simulink model "fft_512pt_co_sim"  (Simulink 8.0)
settings: Solver=ode45  StartTime=0.0  StopTime=1000  RelTol=1e-3
libraries: xbsIndex_r4 x1077
(part 1 of 2)
settings Model: Creator=dell  LastModifiedBy=dell

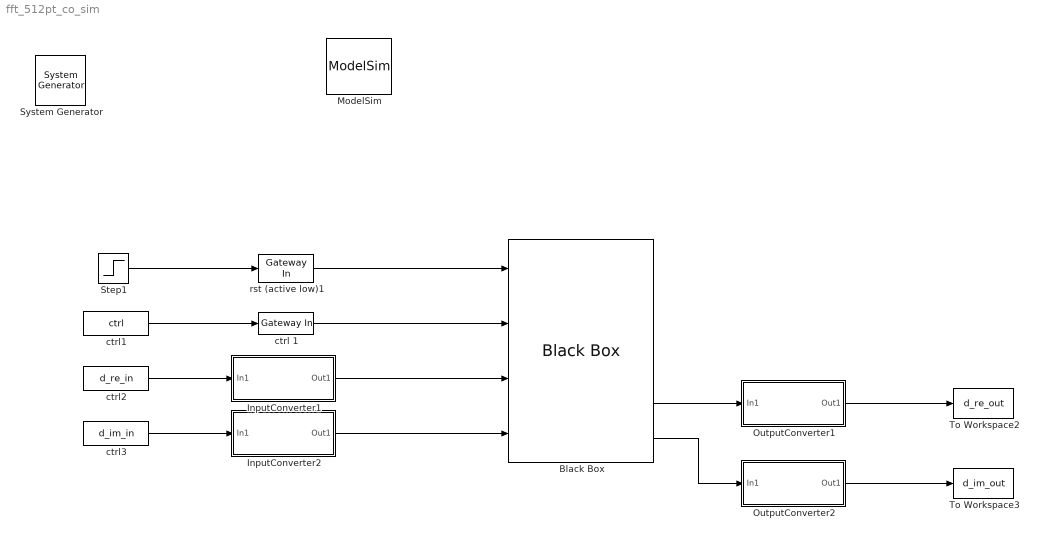
== system fft_512pt_co_sim ==
  " System Generator" : xbsIndex_r4/ System Generator  Tag=genX  xilinxfamily=Kintex7  part=xc7k325t  speed=-3  package=fbg676  synthesis_tool=XST  clock_wrapper=Clock Enables  directory=./netlist  proj_type=Project Navigator  Synth_file=XST Defaults  Impl_file=ISE Defaults  testbench=off  simulink_period=1  sysclk_period=10  dcm_input_clock_period=10  incr_netlist=off  trim_vbits=Everywhere in SubSystem  dbl_ovrd=According to Block Masks  core_generation=According to Block Masks  run_coregen=off  deprecated_control=off  eval_field=0  block_type=sysgen
  Black Box : xbsIndex_r4/Black Box  init_code=fft_pt512_config  sim_method=Inactive  verbose=off  block_type=blackbox2
  InputConverter1 : Subsystem
  InputConverter2 : Subsystem
  ModelSim : xbsIndex_r4/ModelSim  dir=./modelsim  waveform=on  leave_open=on  skip_compile=off  use_unisim=off  use_ver_xilinxcorelib=off  custom_scripts=on  post_vsim_script=./before.do  startup_timeout=40  block_type=hdlcosim
      settings: infoedit="Allow other blocks to schedule HDL co-simulation tasks.<br><br>Note that selecting \"Skip compilation\" when inappropriate can cause simulation errors and failures. Please refer to the block help for details."
  OutputConverter1 : Subsystem
  OutputConverter2 : Subsystem
  Step1 : Step  SampleTime=1
  To Workspace2 : ToWorkspace  VariableName=d_re_out  SampleTime=-1  SaveFormat=Timeseries
  To Workspace3 : ToWorkspace  VariableName=d_im_out  SampleTime=-1  SaveFormat=Timeseries
  ctrl 1 : xbsIndex_r4/Gateway In  gui_display_data_type=Boolean  arith_type=Boolean  n_bits=2  bin_pt=0  preci_type=Single  exp_width=8  frac_width=24  quantization="Round  (unbiased: +/- Inf)"  overflow=Saturate  period=1  dbl_ovrd=off  timing_constraint=None  locs_specified=off  LOCs={}  UseAsADC=off  ADCChannel='1'  inherit_from_input=off  hdl_port=on  block_type=gatewayin
      settings: xl_area=[0, 0, 0, 0, 0, 0, 0]  block_version=VER_STRING_GOES_HERE
  ctrl1 : FromWorkspace  VariableName=ctrl  SampleTime=1
  ctrl2 : FromWorkspace  VariableName=d_re_in  SampleTime=1  Interpolate=off  OutputAfterFinalValue=Setting to zero
  ctrl3 : FromWorkspace  VariableName=d_im_in  SampleTime=1  Interpolate=off  OutputAfterFinalValue=Setting to zero
  rst (active low)1 : xbsIndex_r4/Gateway In  gui_display_data_type=Boolean  arith_type=Boolean  n_bits=10  bin_pt=8  preci_type=Single  exp_width=8  frac_width=24  quantization="Round  (unbiased: +/- Inf)"  overflow=Saturate  period=1  dbl_ovrd=off  timing_constraint=None  locs_specified=off  LOCs={}  UseAsADC=off  ADCChannel='1'  inherit_from_input=off  hdl_port=on  block_type=gatewayin
      settings: xl_area=[0, 0, 0, 0, 0, 0, 0]  block_version=VER_STRING_GOES_HERE
  wires:
  Step1/1 -> rst (active low)1/1
  ctrl1/1 -> ctrl 1/1
  ctrl 1/1 -> Black Box/2
  rst (active low)1/1 -> Black Box/1
  ctrl2/1 -> InputConverter1/1(In1)
  InputConverter1/1(Out1) -> Black Box/3
  ctrl3/1 -> InputConverter2/1(In1)
  InputConverter2/1(Out1) -> Black Box/4
  Black Box/5 -> OutputConverter1/1(In1)
  OutputConverter1/1(Out1) -> To Workspace2/1
  Black Box/6 -> OutputConverter2/1(In1)
  OutputConverter2/1(Out1) -> To Workspace3/1

== system fft_512pt_co_sim/InputConverter1 ==
  In1 : Inport
  Concat : xbsIndex_r4/Concat  num_inputs=8  dbl_ovrd=off  block_type=concat
  Demux : Demux  Outputs=8
  dataconv : Subsystem
  dataconv1 : Subsystem
  dataconv13 : Subsystem
  dataconv26 : Subsystem
  dataconv28 : Subsystem
  dataconv29 : Subsystem
  dataconv3 : Subsystem
  dataconv7 : Subsystem
  Out1 : Outport
  wires:
  Demux/3 -> dataconv26/1(In1)
  Demux/7 -> dataconv28/1(In1)
  Demux/4 -> dataconv7/1(In1)
  Demux/2 -> dataconv29/1(In1)
  Demux/1 -> dataconv/1(In1)
  Demux/5 -> dataconv3/1(In1)
  Demux/6 -> dataconv13/1(In1)
  dataconv/1(Out1) -> Concat/1
  dataconv28/1(Out1) -> Concat/7
  dataconv26/1(Out1) -> Concat/3
  dataconv29/1(Out1) -> Concat/2
  dataconv13/1(Out1) -> Concat/6
  dataconv7/1(Out1) -> Concat/4
  dataconv3/1(Out1) -> Concat/5
  In1/1 -> Demux/1
  Concat/1 -> Out1/1
  Demux/8 -> dataconv1/1(In1)
  dataconv1/1(Out1) -> Concat/8

== system fft_512pt_co_sim/InputConverter2 ==
  In1 : Inport
  Concat : xbsIndex_r4/Concat  num_inputs=8  dbl_ovrd=off  block_type=concat
  Demux : Demux  Outputs=8
  dataconv : Subsystem
  dataconv1 : Subsystem
  dataconv13 : Subsystem
  dataconv26 : Subsystem
  dataconv28 : Subsystem
  dataconv29 : Subsystem
  dataconv3 : Subsystem
  dataconv7 : Subsystem
  Out1 : Outport
  wires:
  Demux/3 -> dataconv26/1(In1)
  Demux/7 -> dataconv28/1(In1)
  Demux/4 -> dataconv7/1(In1)
  Demux/2 -> dataconv29/1(In1)
  Demux/1 -> dataconv/1(In1)
  Demux/5 -> dataconv3/1(In1)
  Demux/6 -> dataconv13/1(In1)
  dataconv/1(Out1) -> Concat/1
  dataconv28/1(Out1) -> Concat/7
  dataconv26/1(Out1) -> Concat/3
  dataconv29/1(Out1) -> Concat/2
  dataconv13/1(Out1) -> Concat/6
  dataconv7/1(Out1) -> Concat/4
  dataconv3/1(Out1) -> Concat/5
  In1/1 -> Demux/1
  Concat/1 -> Out1/1
  Demux/8 -> dataconv1/1(In1)
  dataconv1/1(Out1) -> Concat/8

== system fft_512pt_co_sim/OutputConverter1 ==
  In1 : Inport
  512to64 : Subsystem
  Gateway Out{,1..3,15..18} (8 alike) : xbsIndex_r4/Gateway Out  inherit_from_input=on  hdl_port=on  timing_constraint=None  locs_specified=off  LOCs={}  UseAsDAC=off  DACChannel='1'  block_type=gatewayout
  Mux : Mux  Inputs=8
  Out1 : Outport
  wires:
  In1/1 -> 512to64/1(In1)
  512to64/2(Out3) -> Gateway Out/1
  512to64/1(Out2) -> Gateway Out15/1
  512to64/4(Out5) -> Gateway Out17/1
  512to64/3(Out4) -> Gateway Out16/1
  512to64/5(Out6) -> Gateway Out18/1
  Gateway Out15/1 -> Mux/1
  Gateway Out16/1 -> Mux/3
  Gateway Out17/1 -> Mux/4
  Gateway Out18/1 -> Mux/5
  Gateway Out/1 -> Mux/2
  Mux/1 -> Out1/1
  512to64/6(Out7) -> Gateway Out1/1
  Gateway Out1/1 -> Mux/6
  Gateway Out2/1 -> Mux/7
  512to64/7(Out8) -> Gateway Out2/1
  512to64/8(Out9) -> Gateway Out3/1
  Gateway Out3/1 -> Mux/8

== system fft_512pt_co_sim/OutputConverter2 ==
  In1 : Inport
  512to64 : Subsystem
  Gateway Out{,1..3,15..18} (8 alike) : xbsIndex_r4/Gateway Out  inherit_from_input=on  hdl_port=on  timing_constraint=None  locs_specified=off  LOCs={}  UseAsDAC=off  DACChannel='1'  block_type=gatewayout
  Mux : Mux  Inputs=8
  Out1 : Outport
  wires:
  In1/1 -> 512to64/1(In1)
  512to64/2(Out3) -> Gateway Out/1
  512to64/1(Out2) -> Gateway Out15/1
  512to64/4(Out5) -> Gateway Out17/1
  512to64/3(Out4) -> Gateway Out16/1
  512to64/5(Out6) -> Gateway Out18/1
  Gateway Out15/1 -> Mux/1
  Gateway Out16/1 -> Mux/3
  Gateway Out17/1 -> Mux/4
  Gateway Out18/1 -> Mux/5
  Gateway Out/1 -> Mux/2
  Mux/1 -> Out1/1
  512to64/6(Out7) -> Gateway Out1/1
  Gateway Out1/1 -> Mux/6
  Gateway Out2/1 -> Mux/7
  512to64/7(Out8) -> Gateway Out2/1
  512to64/8(Out9) -> Gateway Out3/1
  Gateway Out3/1 -> Mux/8

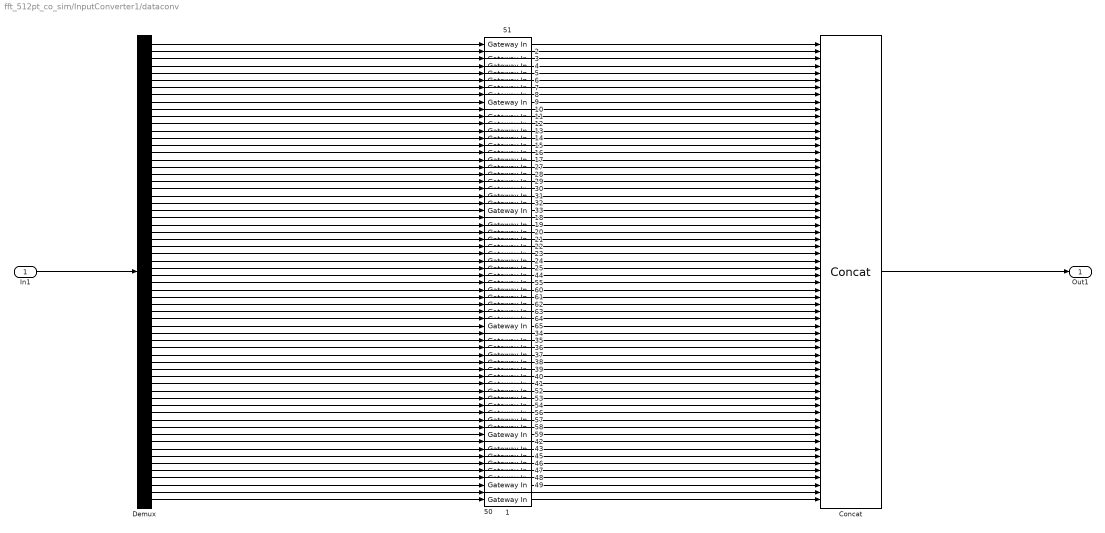
== system fft_512pt_co_sim/InputConverter1/dataconv ==
  In1 : Inport
   {1..25,27..65} (64 alike) : xbsIndex_r4/Gateway In  gui_display_data_type=Boolean  arith_type=Boolean  n_bits=16  bin_pt=14  preci_type=Single  exp_width=8  frac_width=24  quantization="Round  (unbiased: +/- Inf)"  overflow=Saturate  period=1  dbl_ovrd=off  timing_constraint=None  locs_specified=off  LOCs={}  UseAsADC=off  ADCChannel='1'  inherit_from_input=off  hdl_port=on  block_type=gatewayin
  Concat : xbsIndex_r4/Concat  num_inputs=64  dbl_ovrd=off  block_type=concat
  Demux : Demux  Outputs=64
  Out1 : Outport
  wires:
  Demux/12 -> " 12"/1
  Demux/14 -> " 14"/1
  Demux/15 -> " 15"/1
  Demux/17 -> " 17"/1
  Demux/10 -> " 10"/1
  Demux/16 -> " 16"/1
  Demux/18 -> " 27"/1
  Demux/19 -> " 28"/1
  Demux/7 -> " 7"/1
  Demux/20 -> " 29"/1
  Demux/9 -> " 9"/1
  Demux/2 -> " 2"/1
  Demux/13 -> " 13"/1
  Demux/3 -> " 3"/1
  Demux/6 -> " 6"/1
  Demux/11 -> " 11"/1
  Demux/1 -> " 51"/1
  Demux/8 -> " 8"/1
  Demux/4 -> " 4"/1
  Demux/5 -> " 5"/1
  Demux/21 -> " 30"/1
  Demux/25 -> " 18"/1
  Demux/26 -> " 19"/1
  Demux/22 -> " 31"/1
  Demux/30 -> " 23"/1
  Demux/23 -> " 32"/1
  Demux/24 -> " 33"/1
  Demux/27 -> " 20"/1
  Demux/28 -> " 21"/1
  Demux/31 -> " 24"/1
  Demux/32 -> " 25"/1
  Demux/29 -> " 22"/1
  Demux/36 -> " 61"/1
  Demux/34 -> " 55"/1
  Demux/35 -> " 60"/1
  Demux/33 -> " 44"/1
  Demux/49 -> " 52"/1
  Demux/43 -> " 36"/1
  Demux/42 -> " 35"/1
  Demux/44 -> " 37"/1
  Demux/51 -> " 54"/1
  Demux/59 -> " 46"/1
  Demux/60 -> " 47"/1
  Demux/54 -> " 58"/1
  Demux/61 -> " 48"/1
  Demux/47 -> " 40"/1
  Demux/46 -> " 39"/1
  Demux/55 -> " 59"/1
  Demux/39 -> " 64"/1
  Demux/41 -> " 34"/1
  Demux/58 -> " 45"/1
  Demux/52 -> " 56"/1
  Demux/53 -> " 57"/1
  Demux/56 -> " 42"/1
  Demux/57 -> " 43"/1
  Demux/38 -> " 63"/1
  Demux/62 -> " 49"/1
  Demux/50 -> " 53"/1
  Demux/63 -> " 1"/1
  Demux/40 -> " 65"/1
  Demux/48 -> " 41"/1
  Demux/64 -> " 50"/1
  Demux/45 -> " 38"/1
  Demux/37 -> " 62"/1
  " 13"/1 -> Concat/13
  " 11"/1 -> Concat/11
  " 16"/1 -> Concat/16
  " 15"/1 -> Concat/15
  " 10"/1 -> Concat/10
  " 14"/1 -> Concat/14
  " 12"/1 -> Concat/12
  " 17"/1 -> Concat/17
  " 2"/1 -> Concat/2
  " 3"/1 -> Concat/3
  " 7"/1 -> Concat/7
  " 6"/1 -> Concat/6
  " 9"/1 -> Concat/9
  " 8"/1 -> Concat/8
  " 42"/1 -> Concat/56
  " 35"/1 -> Concat/42
  " 43"/1 -> Concat/57
  " 40"/1 -> Concat/47
  " 36"/1 -> Concat/43
  " 34"/1 -> Concat/41
  " 37"/1 -> Concat/44
  " 38"/1 -> Concat/45
  " 41"/1 -> Concat/48
  " 39"/1 -> Concat/46
  " 52"/1 -> Concat/49
  " 56"/1 -> Concat/52
  " 49"/1 -> Concat/62
  " 1"/1 -> Concat/63
  " 44"/1 -> Concat/33
  " 55"/1 -> Concat/34
  " 54"/1 -> Concat/51
  " 53"/1 -> Concat/50
  " 48"/1 -> Concat/61
  " 46"/1 -> Concat/59
  " 45"/1 -> Concat/58
  " 47"/1 -> Concat/60
  " 63"/1 -> Concat/38
  " 62"/1 -> Concat/37
  " 64"/1 -> Concat/39
  " 60"/1 -> Concat/35
  " 65"/1 -> Concat/40
  " 59"/1 -> Concat/55
  " 58"/1 -> Concat/54
  " 57"/1 -> Concat/53
  " 61"/1 -> Concat/36
  " 19"/1 -> Concat/26
  " 20"/1 -> Concat/27
  " 21"/1 -> Concat/28
  " 22"/1 -> Concat/29
  " 23"/1 -> Concat/30
  " 18"/1 -> Concat/25
  " 24"/1 -> Concat/31
  " 25"/1 -> Concat/32
  " 28"/1 -> Concat/19
  " 27"/1 -> Concat/18
  " 30"/1 -> Concat/21
  " 29"/1 -> Concat/20
  " 31"/1 -> Concat/22
  " 32"/1 -> Concat/23
  " 33"/1 -> Concat/24
  " 4"/1 -> Concat/4
  " 5"/1 -> Concat/5
  " 50"/1 -> Concat/64
  " 51"/1 -> Concat/1
  In1/1 -> Demux/1
  Concat/1 -> Out1/1

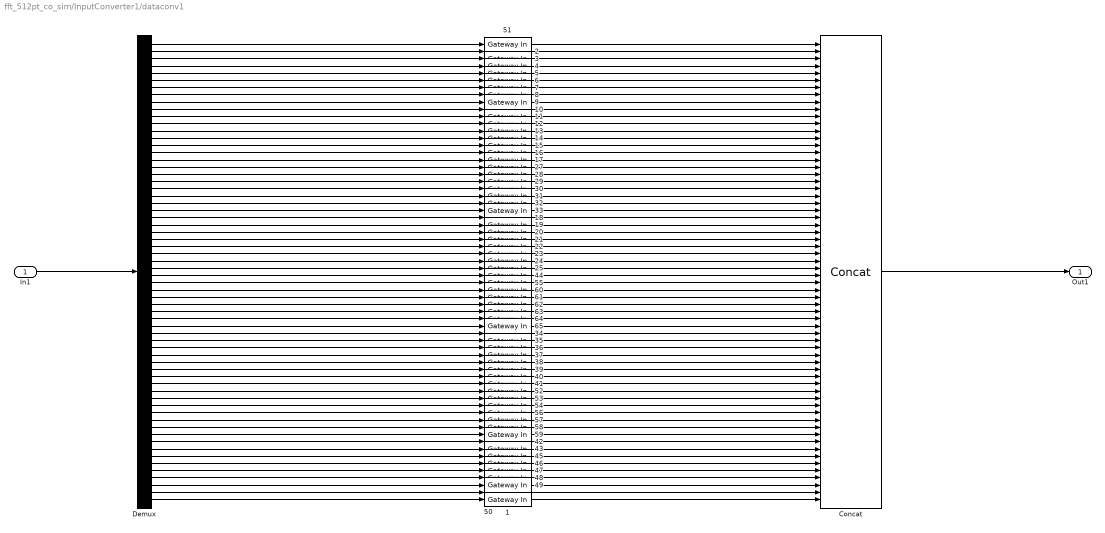
== system fft_512pt_co_sim/InputConverter1/dataconv1 ==
  In1 : Inport
   {1..25,27..65} (64 alike) : xbsIndex_r4/Gateway In  gui_display_data_type=Boolean  arith_type=Boolean  n_bits=16  bin_pt=14  preci_type=Single  exp_width=8  frac_width=24  quantization="Round  (unbiased: +/- Inf)"  overflow=Saturate  period=1  dbl_ovrd=off  timing_constraint=None  locs_specified=off  LOCs={}  UseAsADC=off  ADCChannel='1'  inherit_from_input=off  hdl_port=on  block_type=gatewayin
  Concat : xbsIndex_r4/Concat  num_inputs=64  dbl_ovrd=off  block_type=concat
  Demux : Demux  Outputs=64
  Out1 : Outport
  wires:
  Demux/12 -> " 12"/1
  Demux/14 -> " 14"/1
  Demux/15 -> " 15"/1
  Demux/17 -> " 17"/1
  Demux/10 -> " 10"/1
  Demux/16 -> " 16"/1
  Demux/18 -> " 27"/1
  Demux/19 -> " 28"/1
  Demux/7 -> " 7"/1
  Demux/20 -> " 29"/1
  Demux/9 -> " 9"/1
  Demux/2 -> " 2"/1
  Demux/13 -> " 13"/1
  Demux/3 -> " 3"/1
  Demux/6 -> " 6"/1
  Demux/11 -> " 11"/1
  Demux/1 -> " 51"/1
  Demux/8 -> " 8"/1
  Demux/4 -> " 4"/1
  Demux/5 -> " 5"/1
  Demux/21 -> " 30"/1
  Demux/25 -> " 18"/1
  Demux/26 -> " 19"/1
  Demux/22 -> " 31"/1
  Demux/30 -> " 23"/1
  Demux/23 -> " 32"/1
  Demux/24 -> " 33"/1
  Demux/27 -> " 20"/1
  Demux/28 -> " 21"/1
  Demux/31 -> " 24"/1
  Demux/32 -> " 25"/1
  Demux/29 -> " 22"/1
  Demux/36 -> " 61"/1
  Demux/34 -> " 55"/1
  Demux/35 -> " 60"/1
  Demux/33 -> " 44"/1
  Demux/49 -> " 52"/1
  Demux/43 -> " 36"/1
  Demux/42 -> " 35"/1
  Demux/44 -> " 37"/1
  Demux/51 -> " 54"/1
  Demux/59 -> " 46"/1
  Demux/60 -> " 47"/1
  Demux/54 -> " 58"/1
  Demux/61 -> " 48"/1
  Demux/47 -> " 40"/1
  Demux/46 -> " 39"/1
  Demux/55 -> " 59"/1
  Demux/39 -> " 64"/1
  Demux/41 -> " 34"/1
  Demux/58 -> " 45"/1
  Demux/52 -> " 56"/1
  Demux/53 -> " 57"/1
  Demux/56 -> " 42"/1
  Demux/57 -> " 43"/1
  Demux/38 -> " 63"/1
  Demux/62 -> " 49"/1
  Demux/50 -> " 53"/1
  Demux/63 -> " 1"/1
  Demux/40 -> " 65"/1
  Demux/48 -> " 41"/1
  Demux/64 -> " 50"/1
  Demux/45 -> " 38"/1
  Demux/37 -> " 62"/1
  " 13"/1 -> Concat/13
  " 11"/1 -> Concat/11
  " 16"/1 -> Concat/16
  " 15"/1 -> Concat/15
  " 10"/1 -> Concat/10
  " 14"/1 -> Concat/14
  " 12"/1 -> Concat/12
  " 17"/1 -> Concat/17
  " 2"/1 -> Concat/2
  " 3"/1 -> Concat/3
  " 7"/1 -> Concat/7
  " 6"/1 -> Concat/6
  " 9"/1 -> Concat/9
  " 8"/1 -> Concat/8
  " 42"/1 -> Concat/56
  " 35"/1 -> Concat/42
  " 43"/1 -> Concat/57
  " 40"/1 -> Concat/47
  " 36"/1 -> Concat/43
  " 34"/1 -> Concat/41
  " 37"/1 -> Concat/44
  " 38"/1 -> Concat/45
  " 41"/1 -> Concat/48
  " 39"/1 -> Concat/46
  " 52"/1 -> Concat/49
  " 56"/1 -> Concat/52
  " 49"/1 -> Concat/62
  " 1"/1 -> Concat/63
  " 44"/1 -> Concat/33
  " 55"/1 -> Concat/34
  " 54"/1 -> Concat/51
  " 53"/1 -> Concat/50
  " 48"/1 -> Concat/61
  " 46"/1 -> Concat/59
  " 45"/1 -> Concat/58
  " 47"/1 -> Concat/60
  " 63"/1 -> Concat/38
  " 62"/1 -> Concat/37
  " 64"/1 -> Concat/39
  " 60"/1 -> Concat/35
  " 65"/1 -> Concat/40
  " 59"/1 -> Concat/55
  " 58"/1 -> Concat/54
  " 57"/1 -> Concat/53
  " 61"/1 -> Concat/36
  " 19"/1 -> Concat/26
  " 20"/1 -> Concat/27
  " 21"/1 -> Concat/28
  " 22"/1 -> Concat/29
  " 23"/1 -> Concat/30
  " 18"/1 -> Concat/25
  " 24"/1 -> Concat/31
  " 25"/1 -> Concat/32
  " 28"/1 -> Concat/19
  " 27"/1 -> Concat/18
  " 30"/1 -> Concat/21
  " 29"/1 -> Concat/20
  " 31"/1 -> Concat/22
  " 32"/1 -> Concat/23
  " 33"/1 -> Concat/24
  " 4"/1 -> Concat/4
  " 5"/1 -> Concat/5
  " 50"/1 -> Concat/64
  " 51"/1 -> Concat/1
  In1/1 -> Demux/1
  Concat/1 -> Out1/1

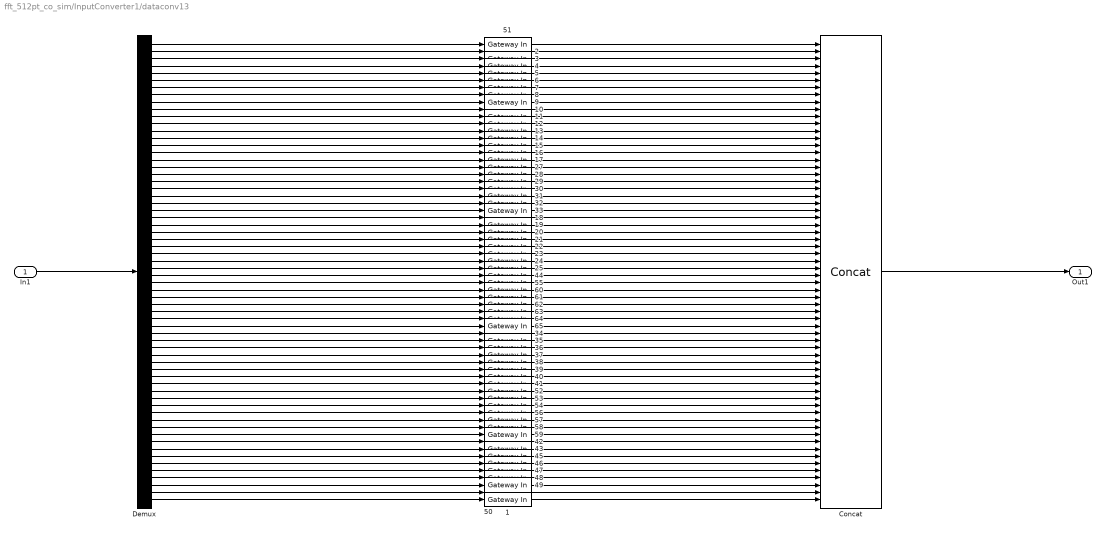
== system fft_512pt_co_sim/InputConverter1/dataconv13 ==
  In1 : Inport
   {1..25,27..65} (64 alike) : xbsIndex_r4/Gateway In  gui_display_data_type=Boolean  arith_type=Boolean  n_bits=16  bin_pt=14  preci_type=Single  exp_width=8  frac_width=24  quantization="Round  (unbiased: +/- Inf)"  overflow=Saturate  period=1  dbl_ovrd=off  timing_constraint=None  locs_specified=off  LOCs={}  UseAsADC=off  ADCChannel='1'  inherit_from_input=off  hdl_port=on  block_type=gatewayin
  Concat : xbsIndex_r4/Concat  num_inputs=64  dbl_ovrd=off  block_type=concat
  Demux : Demux  Outputs=64
  Out1 : Outport
  wires:
  Demux/12 -> " 12"/1
  Demux/14 -> " 14"/1
  Demux/15 -> " 15"/1
  Demux/17 -> " 17"/1
  Demux/10 -> " 10"/1
  Demux/16 -> " 16"/1
  Demux/18 -> " 27"/1
  Demux/19 -> " 28"/1
  Demux/7 -> " 7"/1
  Demux/20 -> " 29"/1
  Demux/9 -> " 9"/1
  Demux/2 -> " 2"/1
  Demux/13 -> " 13"/1
  Demux/3 -> " 3"/1
  Demux/6 -> " 6"/1
  Demux/11 -> " 11"/1
  Demux/1 -> " 51"/1
  Demux/8 -> " 8"/1
  Demux/4 -> " 4"/1
  Demux/5 -> " 5"/1
  Demux/21 -> " 30"/1
  Demux/25 -> " 18"/1
  Demux/26 -> " 19"/1
  Demux/22 -> " 31"/1
  Demux/30 -> " 23"/1
  Demux/23 -> " 32"/1
  Demux/24 -> " 33"/1
  Demux/27 -> " 20"/1
  Demux/28 -> " 21"/1
  Demux/31 -> " 24"/1
  Demux/32 -> " 25"/1
  Demux/29 -> " 22"/1
  Demux/36 -> " 61"/1
  Demux/34 -> " 55"/1
  Demux/35 -> " 60"/1
  Demux/33 -> " 44"/1
  Demux/49 -> " 52"/1
  Demux/43 -> " 36"/1
  Demux/42 -> " 35"/1
  Demux/44 -> " 37"/1
  Demux/51 -> " 54"/1
  Demux/59 -> " 46"/1
  Demux/60 -> " 47"/1
  Demux/54 -> " 58"/1
  Demux/61 -> " 48"/1
  Demux/47 -> " 40"/1
  Demux/46 -> " 39"/1
  Demux/55 -> " 59"/1
  Demux/39 -> " 64"/1
  Demux/41 -> " 34"/1
  Demux/58 -> " 45"/1
  Demux/52 -> " 56"/1
  Demux/53 -> " 57"/1
  Demux/56 -> " 42"/1
  Demux/57 -> " 43"/1
  Demux/38 -> " 63"/1
  Demux/62 -> " 49"/1
  Demux/50 -> " 53"/1
  Demux/63 -> " 1"/1
  Demux/40 -> " 65"/1
  Demux/48 -> " 41"/1
  Demux/64 -> " 50"/1
  Demux/45 -> " 38"/1
  Demux/37 -> " 62"/1
  " 13"/1 -> Concat/13
  " 11"/1 -> Concat/11
  " 16"/1 -> Concat/16
  " 15"/1 -> Concat/15
  " 10"/1 -> Concat/10
  " 14"/1 -> Concat/14
  " 12"/1 -> Concat/12
  " 17"/1 -> Concat/17
  " 2"/1 -> Concat/2
  " 3"/1 -> Concat/3
  " 7"/1 -> Concat/7
  " 6"/1 -> Concat/6
  " 9"/1 -> Concat/9
  " 8"/1 -> Concat/8
  " 42"/1 -> Concat/56
  " 35"/1 -> Concat/42
  " 43"/1 -> Concat/57
  " 40"/1 -> Concat/47
  " 36"/1 -> Concat/43
  " 34"/1 -> Concat/41
  " 37"/1 -> Concat/44
  " 38"/1 -> Concat/45
  " 41"/1 -> Concat/48
  " 39"/1 -> Concat/46
  " 52"/1 -> Concat/49
  " 56"/1 -> Concat/52
  " 49"/1 -> Concat/62
  " 1"/1 -> Concat/63
  " 44"/1 -> Concat/33
  " 55"/1 -> Concat/34
  " 54"/1 -> Concat/51
  " 53"/1 -> Concat/50
  " 48"/1 -> Concat/61
  " 46"/1 -> Concat/59
  " 45"/1 -> Concat/58
  " 47"/1 -> Concat/60
  " 63"/1 -> Concat/38
  " 62"/1 -> Concat/37
  " 64"/1 -> Concat/39
  " 60"/1 -> Concat/35
  " 65"/1 -> Concat/40
  " 59"/1 -> Concat/55
  " 58"/1 -> Concat/54
  " 57"/1 -> Concat/53
  " 61"/1 -> Concat/36
  " 19"/1 -> Concat/26
  " 20"/1 -> Concat/27
  " 21"/1 -> Concat/28
  " 22"/1 -> Concat/29
  " 23"/1 -> Concat/30
  " 18"/1 -> Concat/25
  " 24"/1 -> Concat/31
  " 25"/1 -> Concat/32
  " 28"/1 -> Concat/19
  " 27"/1 -> Concat/18
  " 30"/1 -> Concat/21
  " 29"/1 -> Concat/20
  " 31"/1 -> Concat/22
  " 32"/1 -> Concat/23
  " 33"/1 -> Concat/24
  " 4"/1 -> Concat/4
  " 5"/1 -> Concat/5
  " 50"/1 -> Concat/64
  " 51"/1 -> Concat/1
  In1/1 -> Demux/1
  Concat/1 -> Out1/1

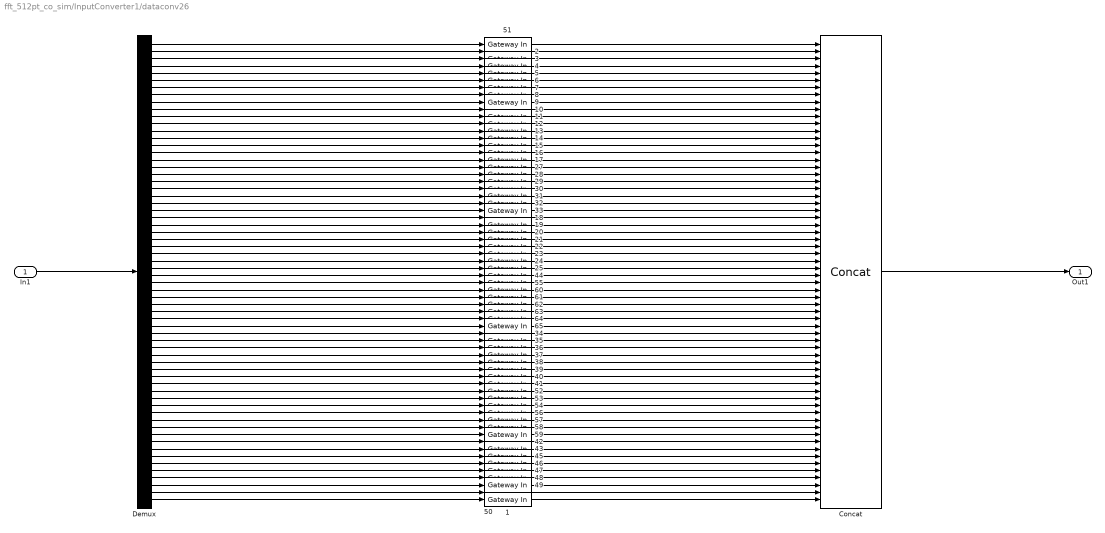
== system fft_512pt_co_sim/InputConverter1/dataconv26 ==
  In1 : Inport
   {1..25,27..65} (64 alike) : xbsIndex_r4/Gateway In  gui_display_data_type=Boolean  arith_type=Boolean  n_bits=16  bin_pt=14  preci_type=Single  exp_width=8  frac_width=24  quantization="Round  (unbiased: +/- Inf)"  overflow=Saturate  period=1  dbl_ovrd=off  timing_constraint=None  locs_specified=off  LOCs={}  UseAsADC=off  ADCChannel='1'  inherit_from_input=off  hdl_port=on  block_type=gatewayin
  Concat : xbsIndex_r4/Concat  num_inputs=64  dbl_ovrd=off  block_type=concat
  Demux : Demux  Outputs=64
  Out1 : Outport
  wires:
  Demux/12 -> " 12"/1
  Demux/14 -> " 14"/1
  Demux/15 -> " 15"/1
  Demux/17 -> " 17"/1
  Demux/10 -> " 10"/1
  Demux/16 -> " 16"/1
  Demux/18 -> " 27"/1
  Demux/19 -> " 28"/1
  Demux/7 -> " 7"/1
  Demux/20 -> " 29"/1
  Demux/9 -> " 9"/1
  Demux/2 -> " 2"/1
  Demux/13 -> " 13"/1
  Demux/3 -> " 3"/1
  Demux/6 -> " 6"/1
  Demux/11 -> " 11"/1
  Demux/1 -> " 51"/1
  Demux/8 -> " 8"/1
  Demux/4 -> " 4"/1
  Demux/5 -> " 5"/1
  Demux/21 -> " 30"/1
  Demux/25 -> " 18"/1
  Demux/26 -> " 19"/1
  Demux/22 -> " 31"/1
  Demux/30 -> " 23"/1
  Demux/23 -> " 32"/1
  Demux/24 -> " 33"/1
  Demux/27 -> " 20"/1
  Demux/28 -> " 21"/1
  Demux/31 -> " 24"/1
  Demux/32 -> " 25"/1
  Demux/29 -> " 22"/1
  Demux/36 -> " 61"/1
  Demux/34 -> " 55"/1
  Demux/35 -> " 60"/1
  Demux/33 -> " 44"/1
  Demux/49 -> " 52"/1
  Demux/43 -> " 36"/1
  Demux/42 -> " 35"/1
  Demux/44 -> " 37"/1
  Demux/51 -> " 54"/1
  Demux/59 -> " 46"/1
  Demux/60 -> " 47"/1
  Demux/54 -> " 58"/1
  Demux/61 -> " 48"/1
  Demux/47 -> " 40"/1
  Demux/46 -> " 39"/1
  Demux/55 -> " 59"/1
  Demux/39 -> " 64"/1
  Demux/41 -> " 34"/1
  Demux/58 -> " 45"/1
  Demux/52 -> " 56"/1
  Demux/53 -> " 57"/1
  Demux/56 -> " 42"/1
  Demux/57 -> " 43"/1
  Demux/38 -> " 63"/1
  Demux/62 -> " 49"/1
  Demux/50 -> " 53"/1
  Demux/63 -> " 1"/1
  Demux/40 -> " 65"/1
  Demux/48 -> " 41"/1
  Demux/64 -> " 50"/1
  Demux/45 -> " 38"/1
  Demux/37 -> " 62"/1
  " 13"/1 -> Concat/13
  " 11"/1 -> Concat/11
  " 16"/1 -> Concat/16
  " 15"/1 -> Concat/15
  " 10"/1 -> Concat/10
  " 14"/1 -> Concat/14
  " 12"/1 -> Concat/12
  " 17"/1 -> Concat/17
  " 2"/1 -> Concat/2
  " 3"/1 -> Concat/3
  " 7"/1 -> Concat/7
  " 6"/1 -> Concat/6
  " 9"/1 -> Concat/9
  " 8"/1 -> Concat/8
  " 42"/1 -> Concat/56
  " 35"/1 -> Concat/42
  " 43"/1 -> Concat/57
  " 40"/1 -> Concat/47
  " 36"/1 -> Concat/43
  " 34"/1 -> Concat/41
  " 37"/1 -> Concat/44
  " 38"/1 -> Concat/45
  " 41"/1 -> Concat/48
  " 39"/1 -> Concat/46
  " 52"/1 -> Concat/49
  " 56"/1 -> Concat/52
  " 49"/1 -> Concat/62
  " 1"/1 -> Concat/63
  " 44"/1 -> Concat/33
  " 55"/1 -> Concat/34
  " 54"/1 -> Concat/51
  " 53"/1 -> Concat/50
  " 48"/1 -> Concat/61
  " 46"/1 -> Concat/59
  " 45"/1 -> Concat/58
  " 47"/1 -> Concat/60
  " 63"/1 -> Concat/38
  " 62"/1 -> Concat/37
  " 64"/1 -> Concat/39
  " 60"/1 -> Concat/35
  " 65"/1 -> Concat/40
  " 59"/1 -> Concat/55
  " 58"/1 -> Concat/54
  " 57"/1 -> Concat/53
  " 61"/1 -> Concat/36
  " 19"/1 -> Concat/26
  " 20"/1 -> Concat/27
  " 21"/1 -> Concat/28
  " 22"/1 -> Concat/29
  " 23"/1 -> Concat/30
  " 18"/1 -> Concat/25
  " 24"/1 -> Concat/31
  " 25"/1 -> Concat/32
  " 28"/1 -> Concat/19
  " 27"/1 -> Concat/18
  " 30"/1 -> Concat/21
  " 29"/1 -> Concat/20
  " 31"/1 -> Concat/22
  " 32"/1 -> Concat/23
  " 33"/1 -> Concat/24
  " 4"/1 -> Concat/4
  " 5"/1 -> Concat/5
  " 50"/1 -> Concat/64
  " 51"/1 -> Concat/1
  In1/1 -> Demux/1
  Concat/1 -> Out1/1

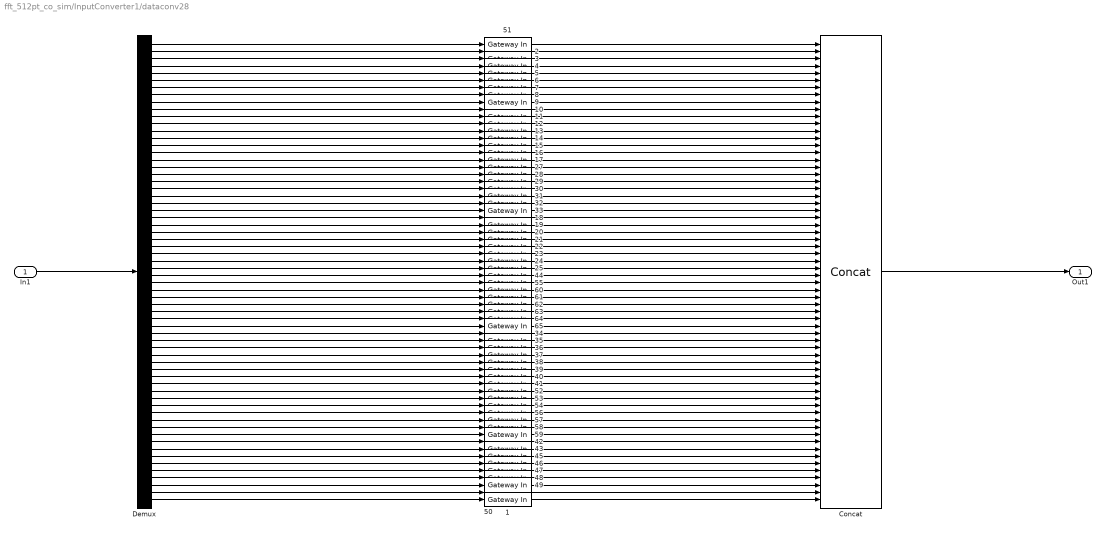
== system fft_512pt_co_sim/InputConverter1/dataconv28 ==
  In1 : Inport
   {1..25,27..65} (64 alike) : xbsIndex_r4/Gateway In  gui_display_data_type=Boolean  arith_type=Boolean  n_bits=16  bin_pt=14  preci_type=Single  exp_width=8  frac_width=24  quantization="Round  (unbiased: +/- Inf)"  overflow=Saturate  period=1  dbl_ovrd=off  timing_constraint=None  locs_specified=off  LOCs={}  UseAsADC=off  ADCChannel='1'  inherit_from_input=off  hdl_port=on  block_type=gatewayin
  Concat : xbsIndex_r4/Concat  num_inputs=64  dbl_ovrd=off  block_type=concat
  Demux : Demux  Outputs=64
  Out1 : Outport
  wires:
  Demux/12 -> " 12"/1
  Demux/14 -> " 14"/1
  Demux/15 -> " 15"/1
  Demux/17 -> " 17"/1
  Demux/10 -> " 10"/1
  Demux/16 -> " 16"/1
  Demux/18 -> " 27"/1
  Demux/19 -> " 28"/1
  Demux/7 -> " 7"/1
  Demux/20 -> " 29"/1
  Demux/9 -> " 9"/1
  Demux/2 -> " 2"/1
  Demux/13 -> " 13"/1
  Demux/3 -> " 3"/1
  Demux/6 -> " 6"/1
  Demux/11 -> " 11"/1
  Demux/1 -> " 51"/1
  Demux/8 -> " 8"/1
  Demux/4 -> " 4"/1
  Demux/5 -> " 5"/1
  Demux/21 -> " 30"/1
  Demux/25 -> " 18"/1
  Demux/26 -> " 19"/1
  Demux/22 -> " 31"/1
  Demux/30 -> " 23"/1
  Demux/23 -> " 32"/1
  Demux/24 -> " 33"/1
  Demux/27 -> " 20"/1
  Demux/28 -> " 21"/1
  Demux/31 -> " 24"/1
  Demux/32 -> " 25"/1
  Demux/29 -> " 22"/1
  Demux/36 -> " 61"/1
  Demux/34 -> " 55"/1
  Demux/35 -> " 60"/1
  Demux/33 -> " 44"/1
  Demux/49 -> " 52"/1
  Demux/43 -> " 36"/1
  Demux/42 -> " 35"/1
  Demux/44 -> " 37"/1
  Demux/51 -> " 54"/1
  Demux/59 -> " 46"/1
  Demux/60 -> " 47"/1
  Demux/54 -> " 58"/1
  Demux/61 -> " 48"/1
  Demux/47 -> " 40"/1
  Demux/46 -> " 39"/1
  Demux/55 -> " 59"/1
  Demux/39 -> " 64"/1
  Demux/41 -> " 34"/1
  Demux/58 -> " 45"/1
  Demux/52 -> " 56"/1
  Demux/53 -> " 57"/1
  Demux/56 -> " 42"/1
  Demux/57 -> " 43"/1
  Demux/38 -> " 63"/1
  Demux/62 -> " 49"/1
  Demux/50 -> " 53"/1
  Demux/63 -> " 1"/1
  Demux/40 -> " 65"/1
  Demux/48 -> " 41"/1
  Demux/64 -> " 50"/1
  Demux/45 -> " 38"/1
  Demux/37 -> " 62"/1
  " 13"/1 -> Concat/13
  " 11"/1 -> Concat/11
  " 16"/1 -> Concat/16
  " 15"/1 -> Concat/15
  " 10"/1 -> Concat/10
  " 14"/1 -> Concat/14
  " 12"/1 -> Concat/12
  " 17"/1 -> Concat/17
  " 2"/1 -> Concat/2
  " 3"/1 -> Concat/3
  " 7"/1 -> Concat/7
  " 6"/1 -> Concat/6
  " 9"/1 -> Concat/9
  " 8"/1 -> Concat/8
  " 42"/1 -> Concat/56
  " 35"/1 -> Concat/42
  " 43"/1 -> Concat/57
  " 40"/1 -> Concat/47
  " 36"/1 -> Concat/43
  " 34"/1 -> Concat/41
  " 37"/1 -> Concat/44
  " 38"/1 -> Concat/45
  " 41"/1 -> Concat/48
  " 39"/1 -> Concat/46
  " 52"/1 -> Concat/49
  " 56"/1 -> Concat/52
  " 49"/1 -> Concat/62
  " 1"/1 -> Concat/63
  " 44"/1 -> Concat/33
  " 55"/1 -> Concat/34
  " 54"/1 -> Concat/51
  " 53"/1 -> Concat/50
  " 48"/1 -> Concat/61
  " 46"/1 -> Concat/59
  " 45"/1 -> Concat/58
  " 47"/1 -> Concat/60
  " 63"/1 -> Concat/38
  " 62"/1 -> Concat/37
  " 64"/1 -> Concat/39
  " 60"/1 -> Concat/35
  " 65"/1 -> Concat/40
  " 59"/1 -> Concat/55
  " 58"/1 -> Concat/54
  " 57"/1 -> Concat/53
  " 61"/1 -> Concat/36
  " 19"/1 -> Concat/26
  " 20"/1 -> Concat/27
  " 21"/1 -> Concat/28
  " 22"/1 -> Concat/29
  " 23"/1 -> Concat/30
  " 18"/1 -> Concat/25
  " 24"/1 -> Concat/31
  " 25"/1 -> Concat/32
  " 28"/1 -> Concat/19
  " 27"/1 -> Concat/18
  " 30"/1 -> Concat/21
  " 29"/1 -> Concat/20
  " 31"/1 -> Concat/22
  " 32"/1 -> Concat/23
  " 33"/1 -> Concat/24
  " 4"/1 -> Concat/4
  " 5"/1 -> Concat/5
  " 50"/1 -> Concat/64
  " 51"/1 -> Concat/1
  In1/1 -> Demux/1
  Concat/1 -> Out1/1

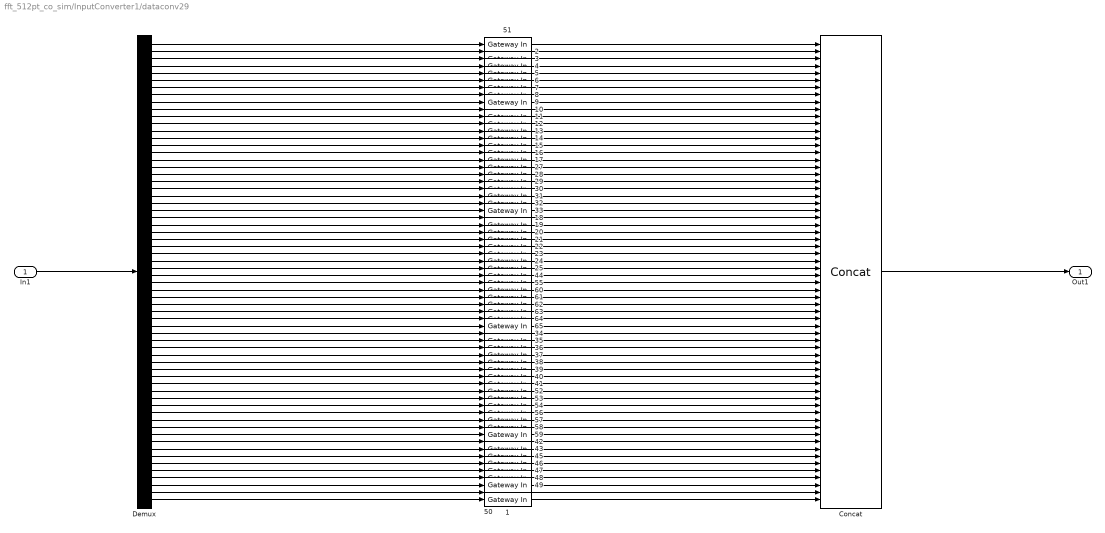
== system fft_512pt_co_sim/InputConverter1/dataconv29 ==
  In1 : Inport
   {1..25,27..65} (64 alike) : xbsIndex_r4/Gateway In  gui_display_data_type=Boolean  arith_type=Boolean  n_bits=16  bin_pt=14  preci_type=Single  exp_width=8  frac_width=24  quantization="Round  (unbiased: +/- Inf)"  overflow=Saturate  period=1  dbl_ovrd=off  timing_constraint=None  locs_specified=off  LOCs={}  UseAsADC=off  ADCChannel='1'  inherit_from_input=off  hdl_port=on  block_type=gatewayin
  Concat : xbsIndex_r4/Concat  num_inputs=64  dbl_ovrd=off  block_type=concat
  Demux : Demux  Outputs=64
  Out1 : Outport
  wires:
  Demux/12 -> " 12"/1
  Demux/14 -> " 14"/1
  Demux/15 -> " 15"/1
  Demux/17 -> " 17"/1
  Demux/10 -> " 10"/1
  Demux/16 -> " 16"/1
  Demux/18 -> " 27"/1
  Demux/19 -> " 28"/1
  Demux/7 -> " 7"/1
  Demux/20 -> " 29"/1
  Demux/9 -> " 9"/1
  Demux/2 -> " 2"/1
  Demux/13 -> " 13"/1
  Demux/3 -> " 3"/1
  Demux/6 -> " 6"/1
  Demux/11 -> " 11"/1
  Demux/1 -> " 51"/1
  Demux/8 -> " 8"/1
  Demux/4 -> " 4"/1
  Demux/5 -> " 5"/1
  Demux/21 -> " 30"/1
  Demux/25 -> " 18"/1
  Demux/26 -> " 19"/1
  Demux/22 -> " 31"/1
  Demux/30 -> " 23"/1
  Demux/23 -> " 32"/1
  Demux/24 -> " 33"/1
  Demux/27 -> " 20"/1
  Demux/28 -> " 21"/1
  Demux/31 -> " 24"/1
  Demux/32 -> " 25"/1
  Demux/29 -> " 22"/1
  Demux/36 -> " 61"/1
  Demux/34 -> " 55"/1
  Demux/35 -> " 60"/1
  Demux/33 -> " 44"/1
  Demux/49 -> " 52"/1
  Demux/43 -> " 36"/1
  Demux/42 -> " 35"/1
  Demux/44 -> " 37"/1
  Demux/51 -> " 54"/1
  Demux/59 -> " 46"/1
  Demux/60 -> " 47"/1
  Demux/54 -> " 58"/1
  Demux/61 -> " 48"/1
  Demux/47 -> " 40"/1
  Demux/46 -> " 39"/1
  Demux/55 -> " 59"/1
  Demux/39 -> " 64"/1
  Demux/41 -> " 34"/1
  Demux/58 -> " 45"/1
  Demux/52 -> " 56"/1
  Demux/53 -> " 57"/1
  Demux/56 -> " 42"/1
  Demux/57 -> " 43"/1
  Demux/38 -> " 63"/1
  Demux/62 -> " 49"/1
  Demux/50 -> " 53"/1
  Demux/63 -> " 1"/1
  Demux/40 -> " 65"/1
  Demux/48 -> " 41"/1
  Demux/64 -> " 50"/1
  Demux/45 -> " 38"/1
  Demux/37 -> " 62"/1
  " 13"/1 -> Concat/13
  " 11"/1 -> Concat/11
  " 16"/1 -> Concat/16
  " 15"/1 -> Concat/15
  " 10"/1 -> Concat/10
  " 14"/1 -> Concat/14
  " 12"/1 -> Concat/12
  " 17"/1 -> Concat/17
  " 2"/1 -> Concat/2
  " 3"/1 -> Concat/3
  " 7"/1 -> Concat/7
  " 6"/1 -> Concat/6
  " 9"/1 -> Concat/9
  " 8"/1 -> Concat/8
  " 42"/1 -> Concat/56
  " 35"/1 -> Concat/42
  " 43"/1 -> Concat/57
  " 40"/1 -> Concat/47
  " 36"/1 -> Concat/43
  " 34"/1 -> Concat/41
  " 37"/1 -> Concat/44
  " 38"/1 -> Concat/45
  " 41"/1 -> Concat/48
  " 39"/1 -> Concat/46
  " 52"/1 -> Concat/49
  " 56"/1 -> Concat/52
  " 49"/1 -> Concat/62
  " 1"/1 -> Concat/63
  " 44"/1 -> Concat/33
  " 55"/1 -> Concat/34
  " 54"/1 -> Concat/51
  " 53"/1 -> Concat/50
  " 48"/1 -> Concat/61
  " 46"/1 -> Concat/59
  " 45"/1 -> Concat/58
  " 47"/1 -> Concat/60
  " 63"/1 -> Concat/38
  " 62"/1 -> Concat/37
  " 64"/1 -> Concat/39
  " 60"/1 -> Concat/35
  " 65"/1 -> Concat/40
  " 59"/1 -> Concat/55
  " 58"/1 -> Concat/54
  " 57"/1 -> Concat/53
  " 61"/1 -> Concat/36
  " 19"/1 -> Concat/26
  " 20"/1 -> Concat/27
  " 21"/1 -> Concat/28
  " 22"/1 -> Concat/29
  " 23"/1 -> Concat/30
  " 18"/1 -> Concat/25
  " 24"/1 -> Concat/31
  " 25"/1 -> Concat/32
  " 28"/1 -> Concat/19
  " 27"/1 -> Concat/18
  " 30"/1 -> Concat/21
  " 29"/1 -> Concat/20
  " 31"/1 -> Concat/22
  " 32"/1 -> Concat/23
  " 33"/1 -> Concat/24
  " 4"/1 -> Concat/4
  " 5"/1 -> Concat/5
  " 50"/1 -> Concat/64
  " 51"/1 -> Concat/1
  In1/1 -> Demux/1
  Concat/1 -> Out1/1

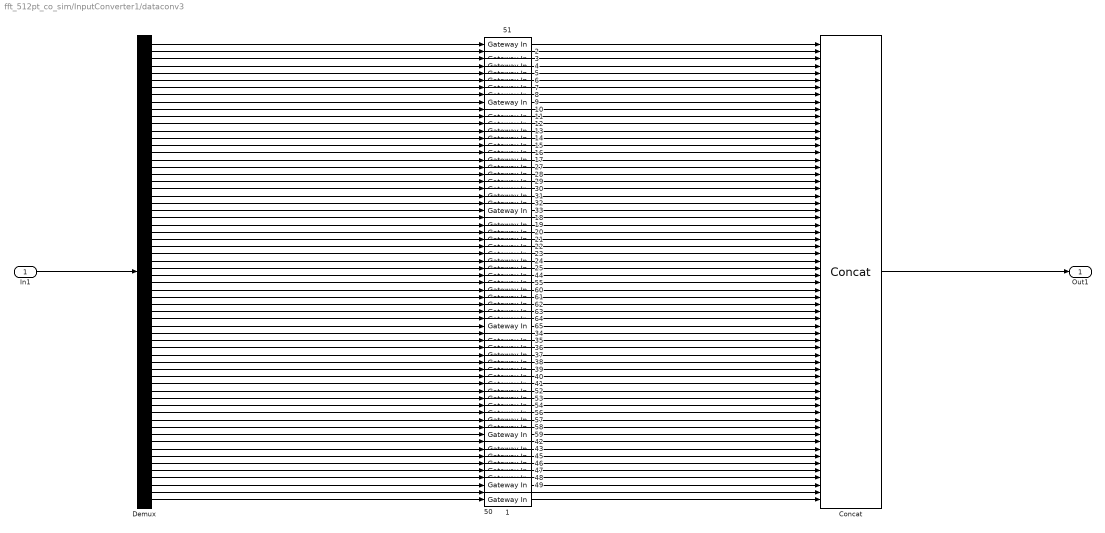
== system fft_512pt_co_sim/InputConverter1/dataconv3 ==
  In1 : Inport
   {1..25,27..65} (64 alike) : xbsIndex_r4/Gateway In  gui_display_data_type=Boolean  arith_type=Boolean  n_bits=16  bin_pt=14  preci_type=Single  exp_width=8  frac_width=24  quantization="Round  (unbiased: +/- Inf)"  overflow=Saturate  period=1  dbl_ovrd=off  timing_constraint=None  locs_specified=off  LOCs={}  UseAsADC=off  ADCChannel='1'  inherit_from_input=off  hdl_port=on  block_type=gatewayin
  Concat : xbsIndex_r4/Concat  num_inputs=64  dbl_ovrd=off  block_type=concat
  Demux : Demux  Outputs=64
  Out1 : Outport
  wires:
  Demux/12 -> " 12"/1
  Demux/14 -> " 14"/1
  Demux/15 -> " 15"/1
  Demux/17 -> " 17"/1
  Demux/10 -> " 10"/1
  Demux/16 -> " 16"/1
  Demux/18 -> " 27"/1
  Demux/19 -> " 28"/1
  Demux/7 -> " 7"/1
  Demux/20 -> " 29"/1
  Demux/9 -> " 9"/1
  Demux/2 -> " 2"/1
  Demux/13 -> " 13"/1
  Demux/3 -> " 3"/1
  Demux/6 -> " 6"/1
  Demux/11 -> " 11"/1
  Demux/1 -> " 51"/1
  Demux/8 -> " 8"/1
  Demux/4 -> " 4"/1
  Demux/5 -> " 5"/1
  Demux/21 -> " 30"/1
  Demux/25 -> " 18"/1
  Demux/26 -> " 19"/1
  Demux/22 -> " 31"/1
  Demux/30 -> " 23"/1
  Demux/23 -> " 32"/1
  Demux/24 -> " 33"/1
  Demux/27 -> " 20"/1
  Demux/28 -> " 21"/1
  Demux/31 -> " 24"/1
  Demux/32 -> " 25"/1
  Demux/29 -> " 22"/1
  Demux/36 -> " 61"/1
  Demux/34 -> " 55"/1
  Demux/35 -> " 60"/1
  Demux/33 -> " 44"/1
  Demux/49 -> " 52"/1
  Demux/43 -> " 36"/1
  Demux/42 -> " 35"/1
  Demux/44 -> " 37"/1
  Demux/51 -> " 54"/1
  Demux/59 -> " 46"/1
  Demux/60 -> " 47"/1
  Demux/54 -> " 58"/1
  Demux/61 -> " 48"/1
  Demux/47 -> " 40"/1
  Demux/46 -> " 39"/1
  Demux/55 -> " 59"/1
  Demux/39 -> " 64"/1
  Demux/41 -> " 34"/1
  Demux/58 -> " 45"/1
  Demux/52 -> " 56"/1
  Demux/53 -> " 57"/1
  Demux/56 -> " 42"/1
  Demux/57 -> " 43"/1
  Demux/38 -> " 63"/1
  Demux/62 -> " 49"/1
  Demux/50 -> " 53"/1
  Demux/63 -> " 1"/1
  Demux/40 -> " 65"/1
  Demux/48 -> " 41"/1
  Demux/64 -> " 50"/1
  Demux/45 -> " 38"/1
  Demux/37 -> " 62"/1
  " 13"/1 -> Concat/13
  " 11"/1 -> Concat/11
  " 16"/1 -> Concat/16
  " 15"/1 -> Concat/15
  " 10"/1 -> Concat/10
  " 14"/1 -> Concat/14
  " 12"/1 -> Concat/12
  " 17"/1 -> Concat/17
  " 2"/1 -> Concat/2
  " 3"/1 -> Concat/3
  " 7"/1 -> Concat/7
  " 6"/1 -> Concat/6
  " 9"/1 -> Concat/9
  " 8"/1 -> Concat/8
  " 42"/1 -> Concat/56
  " 35"/1 -> Concat/42
  " 43"/1 -> Concat/57
  " 40"/1 -> Concat/47
  " 36"/1 -> Concat/43
  " 34"/1 -> Concat/41
  " 37"/1 -> Concat/44
  " 38"/1 -> Concat/45
  " 41"/1 -> Concat/48
  " 39"/1 -> Concat/46
  " 52"/1 -> Concat/49
  " 56"/1 -> Concat/52
  " 49"/1 -> Concat/62
  " 1"/1 -> Concat/63
  " 44"/1 -> Concat/33
  " 55"/1 -> Concat/34
  " 54"/1 -> Concat/51
  " 53"/1 -> Concat/50
  " 48"/1 -> Concat/61
  " 46"/1 -> Concat/59
  " 45"/1 -> Concat/58
  " 47"/1 -> Concat/60
  " 63"/1 -> Concat/38
  " 62"/1 -> Concat/37
  " 64"/1 -> Concat/39
  " 60"/1 -> Concat/35
  " 65"/1 -> Concat/40
  " 59"/1 -> Concat/55
  " 58"/1 -> Concat/54
  " 57"/1 -> Concat/53
  " 61"/1 -> Concat/36
  " 19"/1 -> Concat/26
  " 20"/1 -> Concat/27
  " 21"/1 -> Concat/28
  " 22"/1 -> Concat/29
  " 23"/1 -> Concat/30
  " 18"/1 -> Concat/25
  " 24"/1 -> Concat/31
  " 25"/1 -> Concat/32
  " 28"/1 -> Concat/19
  " 27"/1 -> Concat/18
  " 30"/1 -> Concat/21
  " 29"/1 -> Concat/20
  " 31"/1 -> Concat/22
  " 32"/1 -> Concat/23
  " 33"/1 -> Concat/24
  " 4"/1 -> Concat/4
  " 5"/1 -> Concat/5
  " 50"/1 -> Concat/64
  " 51"/1 -> Concat/1
  In1/1 -> Demux/1
  Concat/1 -> Out1/1

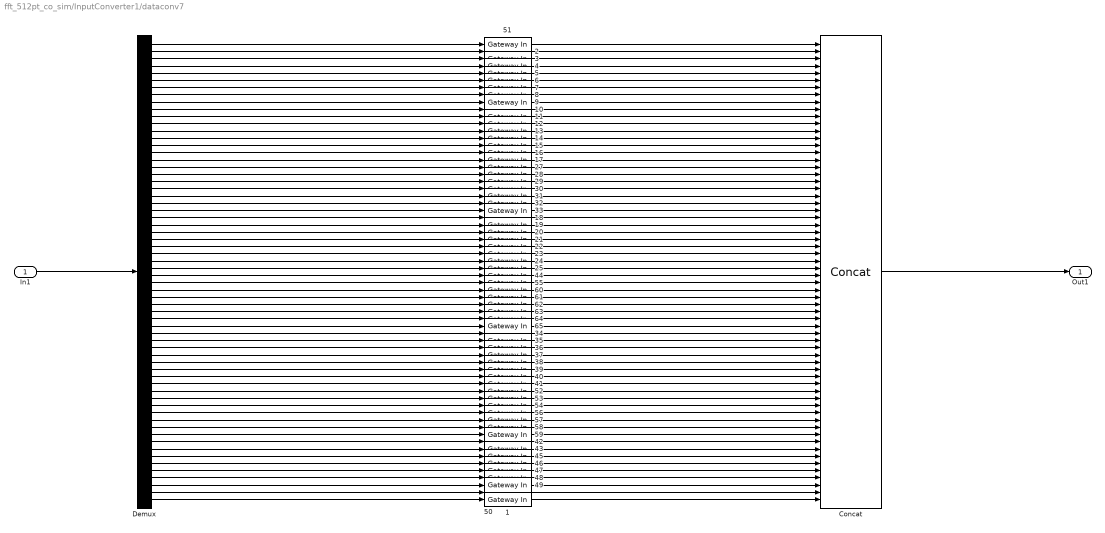
== system fft_512pt_co_sim/InputConverter1/dataconv7 ==
  In1 : Inport
   {1..25,27..65} (64 alike) : xbsIndex_r4/Gateway In  gui_display_data_type=Boolean  arith_type=Boolean  n_bits=16  bin_pt=14  preci_type=Single  exp_width=8  frac_width=24  quantization="Round  (unbiased: +/- Inf)"  overflow=Saturate  period=1  dbl_ovrd=off  timing_constraint=None  locs_specified=off  LOCs={}  UseAsADC=off  ADCChannel='1'  inherit_from_input=off  hdl_port=on  block_type=gatewayin
  Concat : xbsIndex_r4/Concat  num_inputs=64  dbl_ovrd=off  block_type=concat
  Demux : Demux  Outputs=64
  Out1 : Outport
  wires:
  Demux/12 -> " 12"/1
  Demux/14 -> " 14"/1
  Demux/15 -> " 15"/1
  Demux/17 -> " 17"/1
  Demux/10 -> " 10"/1
  Demux/16 -> " 16"/1
  Demux/18 -> " 27"/1
  Demux/19 -> " 28"/1
  Demux/7 -> " 7"/1
  Demux/20 -> " 29"/1
  Demux/9 -> " 9"/1
  Demux/2 -> " 2"/1
  Demux/13 -> " 13"/1
  Demux/3 -> " 3"/1
  Demux/6 -> " 6"/1
  Demux/11 -> " 11"/1
  Demux/1 -> " 51"/1
  Demux/8 -> " 8"/1
  Demux/4 -> " 4"/1
  Demux/5 -> " 5"/1
  Demux/21 -> " 30"/1
  Demux/25 -> " 18"/1
  Demux/26 -> " 19"/1
  Demux/22 -> " 31"/1
  Demux/30 -> " 23"/1
  Demux/23 -> " 32"/1
  Demux/24 -> " 33"/1
  Demux/27 -> " 20"/1
  Demux/28 -> " 21"/1
  Demux/31 -> " 24"/1
  Demux/32 -> " 25"/1
  Demux/29 -> " 22"/1
  Demux/36 -> " 61"/1
  Demux/34 -> " 55"/1
  Demux/35 -> " 60"/1
  Demux/33 -> " 44"/1
  Demux/49 -> " 52"/1
  Demux/43 -> " 36"/1
  Demux/42 -> " 35"/1
  Demux/44 -> " 37"/1
  Demux/51 -> " 54"/1
  Demux/59 -> " 46"/1
  Demux/60 -> " 47"/1
  Demux/54 -> " 58"/1
  Demux/61 -> " 48"/1
  Demux/47 -> " 40"/1
  Demux/46 -> " 39"/1
  Demux/55 -> " 59"/1
  Demux/39 -> " 64"/1
  Demux/41 -> " 34"/1
  Demux/58 -> " 45"/1
  Demux/52 -> " 56"/1
  Demux/53 -> " 57"/1
  Demux/56 -> " 42"/1
  Demux/57 -> " 43"/1
  Demux/38 -> " 63"/1
  Demux/62 -> " 49"/1
  Demux/50 -> " 53"/1
  Demux/63 -> " 1"/1
  Demux/40 -> " 65"/1
  Demux/48 -> " 41"/1
  Demux/64 -> " 50"/1
  Demux/45 -> " 38"/1
  Demux/37 -> " 62"/1
  " 13"/1 -> Concat/13
  " 11"/1 -> Concat/11
  " 16"/1 -> Concat/16
  " 15"/1 -> Concat/15
  " 10"/1 -> Concat/10
  " 14"/1 -> Concat/14
  " 12"/1 -> Concat/12
  " 17"/1 -> Concat/17
  " 2"/1 -> Concat/2
  " 3"/1 -> Concat/3
  " 7"/1 -> Concat/7
  " 6"/1 -> Concat/6
  " 9"/1 -> Concat/9
  " 8"/1 -> Concat/8
  " 42"/1 -> Concat/56
  " 35"/1 -> Concat/42
  " 43"/1 -> Concat/57
  " 40"/1 -> Concat/47
  " 36"/1 -> Concat/43
  " 34"/1 -> Concat/41
  " 37"/1 -> Concat/44
  " 38"/1 -> Concat/45
  " 41"/1 -> Concat/48
  " 39"/1 -> Concat/46
  " 52"/1 -> Concat/49
  " 56"/1 -> Concat/52
  " 49"/1 -> Concat/62
  " 1"/1 -> Concat/63
  " 44"/1 -> Concat/33
  " 55"/1 -> Concat/34
  " 54"/1 -> Concat/51
  " 53"/1 -> Concat/50
  " 48"/1 -> Concat/61
  " 46"/1 -> Concat/59
  " 45"/1 -> Concat/58
  " 47"/1 -> Concat/60
  " 63"/1 -> Concat/38
  " 62"/1 -> Concat/37
  " 64"/1 -> Concat/39
  " 60"/1 -> Concat/35
  " 65"/1 -> Concat/40
  " 59"/1 -> Concat/55
  " 58"/1 -> Concat/54
  " 57"/1 -> Concat/53
  " 61"/1 -> Concat/36
  " 19"/1 -> Concat/26
  " 20"/1 -> Concat/27
  " 21"/1 -> Concat/28
  " 22"/1 -> Concat/29
  " 23"/1 -> Concat/30
  " 18"/1 -> Concat/25
  " 24"/1 -> Concat/31
  " 25"/1 -> Concat/32
  " 28"/1 -> Concat/19
  " 27"/1 -> Concat/18
  " 30"/1 -> Concat/21
  " 29"/1 -> Concat/20
  " 31"/1 -> Concat/22
  " 32"/1 -> Concat/23
  " 33"/1 -> Concat/24
  " 4"/1 -> Concat/4
  " 5"/1 -> Concat/5
  " 50"/1 -> Concat/64
  " 51"/1 -> Concat/1
  In1/1 -> Demux/1
  Concat/1 -> Out1/1

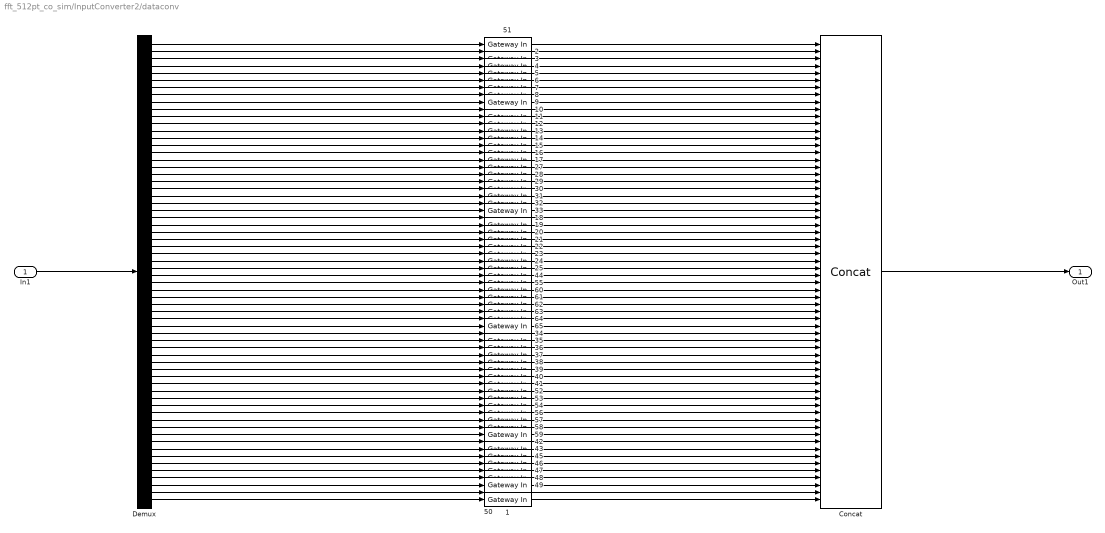
== system fft_512pt_co_sim/InputConverter2/dataconv ==
  In1 : Inport
   {1..25,27..65} (64 alike) : xbsIndex_r4/Gateway In  gui_display_data_type=Boolean  arith_type=Boolean  n_bits=16  bin_pt=14  preci_type=Single  exp_width=8  frac_width=24  quantization="Round  (unbiased: +/- Inf)"  overflow=Saturate  period=1  dbl_ovrd=off  timing_constraint=None  locs_specified=off  LOCs={}  UseAsADC=off  ADCChannel='1'  inherit_from_input=off  hdl_port=on  block_type=gatewayin
  Concat : xbsIndex_r4/Concat  num_inputs=64  dbl_ovrd=off  block_type=concat
  Demux : Demux  Outputs=64
  Out1 : Outport
  wires:
  Demux/12 -> " 12"/1
  Demux/14 -> " 14"/1
  Demux/15 -> " 15"/1
  Demux/17 -> " 17"/1
  Demux/10 -> " 10"/1
  Demux/16 -> " 16"/1
  Demux/18 -> " 27"/1
  Demux/19 -> " 28"/1
  Demux/7 -> " 7"/1
  Demux/20 -> " 29"/1
  Demux/9 -> " 9"/1
  Demux/2 -> " 2"/1
  Demux/13 -> " 13"/1
  Demux/3 -> " 3"/1
  Demux/6 -> " 6"/1
  Demux/11 -> " 11"/1
  Demux/1 -> " 51"/1
  Demux/8 -> " 8"/1
  Demux/4 -> " 4"/1
  Demux/5 -> " 5"/1
  Demux/21 -> " 30"/1
  Demux/25 -> " 18"/1
  Demux/26 -> " 19"/1
  Demux/22 -> " 31"/1
  Demux/30 -> " 23"/1
  Demux/23 -> " 32"/1
  Demux/24 -> " 33"/1
  Demux/27 -> " 20"/1
  Demux/28 -> " 21"/1
  Demux/31 -> " 24"/1
  Demux/32 -> " 25"/1
  Demux/29 -> " 22"/1
  Demux/36 -> " 61"/1
  Demux/34 -> " 55"/1
  Demux/35 -> " 60"/1
  Demux/33 -> " 44"/1
  Demux/49 -> " 52"/1
  Demux/43 -> " 36"/1
  Demux/42 -> " 35"/1
  Demux/44 -> " 37"/1
  Demux/51 -> " 54"/1
  Demux/59 -> " 46"/1
  Demux/60 -> " 47"/1
  Demux/54 -> " 58"/1
  Demux/61 -> " 48"/1
  Demux/47 -> " 40"/1
  Demux/46 -> " 39"/1
  Demux/55 -> " 59"/1
  Demux/39 -> " 64"/1
  Demux/41 -> " 34"/1
  Demux/58 -> " 45"/1
  Demux/52 -> " 56"/1
  Demux/53 -> " 57"/1
  Demux/56 -> " 42"/1
  Demux/57 -> " 43"/1
  Demux/38 -> " 63"/1
  Demux/62 -> " 49"/1
  Demux/50 -> " 53"/1
  Demux/63 -> " 1"/1
  Demux/40 -> " 65"/1
  Demux/48 -> " 41"/1
  Demux/64 -> " 50"/1
  Demux/45 -> " 38"/1
  Demux/37 -> " 62"/1
  " 13"/1 -> Concat/13
  " 11"/1 -> Concat/11
  " 16"/1 -> Concat/16
  " 15"/1 -> Concat/15
  " 10"/1 -> Concat/10
  " 14"/1 -> Concat/14
  " 12"/1 -> Concat/12
  " 17"/1 -> Concat/17
  " 2"/1 -> Concat/2
  " 3"/1 -> Concat/3
  " 7"/1 -> Concat/7
  " 6"/1 -> Concat/6
  " 9"/1 -> Concat/9
  " 8"/1 -> Concat/8
  " 42"/1 -> Concat/56
  " 35"/1 -> Concat/42
  " 43"/1 -> Concat/57
  " 40"/1 -> Concat/47
  " 36"/1 -> Concat/43
  " 34"/1 -> Concat/41
  " 37"/1 -> Concat/44
  " 38"/1 -> Concat/45
  " 41"/1 -> Concat/48
  " 39"/1 -> Concat/46
  " 52"/1 -> Concat/49
  " 56"/1 -> Concat/52
  " 49"/1 -> Concat/62
  " 1"/1 -> Concat/63
  " 44"/1 -> Concat/33
  " 55"/1 -> Concat/34
  " 54"/1 -> Concat/51
  " 53"/1 -> Concat/50
  " 48"/1 -> Concat/61
  " 46"/1 -> Concat/59
  " 45"/1 -> Concat/58
  " 47"/1 -> Concat/60
  " 63"/1 -> Concat/38
  " 62"/1 -> Concat/37
  " 64"/1 -> Concat/39
  " 60"/1 -> Concat/35
  " 65"/1 -> Concat/40
  " 59"/1 -> Concat/55
  " 58"/1 -> Concat/54
  " 57"/1 -> Concat/53
  " 61"/1 -> Concat/36
  " 19"/1 -> Concat/26
  " 20"/1 -> Concat/27
  " 21"/1 -> Concat/28
  " 22"/1 -> Concat/29
  " 23"/1 -> Concat/30
  " 18"/1 -> Concat/25
  " 24"/1 -> Concat/31
  " 25"/1 -> Concat/32
  " 28"/1 -> Concat/19
  " 27"/1 -> Concat/18
  " 30"/1 -> Concat/21
  " 29"/1 -> Concat/20
  " 31"/1 -> Concat/22
  " 32"/1 -> Concat/23
  " 33"/1 -> Concat/24
  " 4"/1 -> Concat/4
  " 5"/1 -> Concat/5
  " 50"/1 -> Concat/64
  " 51"/1 -> Concat/1
  In1/1 -> Demux/1
  Concat/1 -> Out1/1

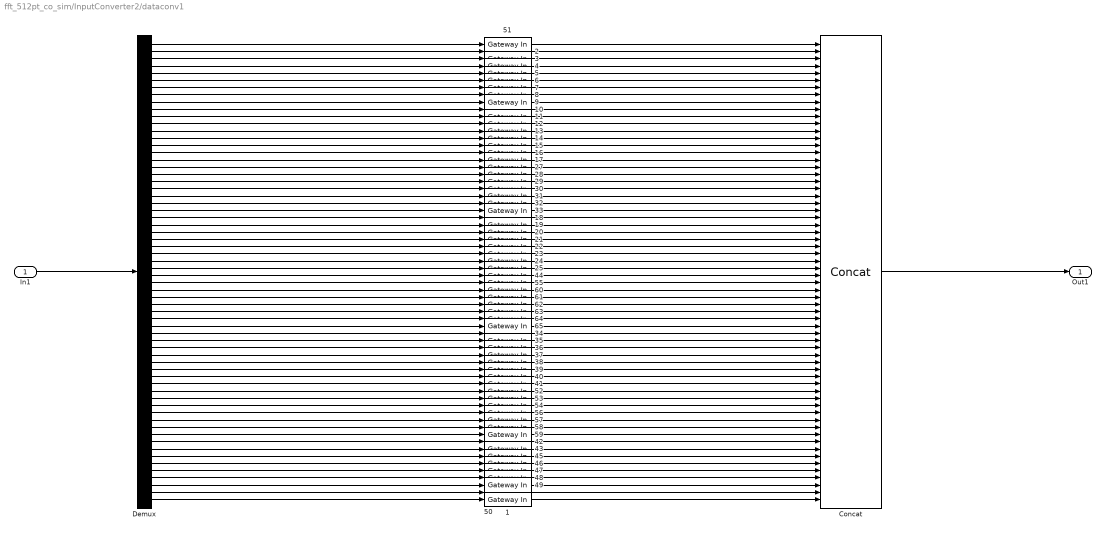
== system fft_512pt_co_sim/InputConverter2/dataconv1 ==
  In1 : Inport
   {1..25,27..65} (64 alike) : xbsIndex_r4/Gateway In  gui_display_data_type=Boolean  arith_type=Boolean  n_bits=16  bin_pt=14  preci_type=Single  exp_width=8  frac_width=24  quantization="Round  (unbiased: +/- Inf)"  overflow=Saturate  period=1  dbl_ovrd=off  timing_constraint=None  locs_specified=off  LOCs={}  UseAsADC=off  ADCChannel='1'  inherit_from_input=off  hdl_port=on  block_type=gatewayin
  Concat : xbsIndex_r4/Concat  num_inputs=64  dbl_ovrd=off  block_type=concat
  Demux : Demux  Outputs=64
  Out1 : Outport
  wires:
  Demux/12 -> " 12"/1
  Demux/14 -> " 14"/1
  Demux/15 -> " 15"/1
  Demux/17 -> " 17"/1
  Demux/10 -> " 10"/1
  Demux/16 -> " 16"/1
  Demux/18 -> " 27"/1
  Demux/19 -> " 28"/1
  Demux/7 -> " 7"/1
  Demux/20 -> " 29"/1
  Demux/9 -> " 9"/1
  Demux/2 -> " 2"/1
  Demux/13 -> " 13"/1
  Demux/3 -> " 3"/1
  Demux/6 -> " 6"/1
  Demux/11 -> " 11"/1
  Demux/1 -> " 51"/1
  Demux/8 -> " 8"/1
  Demux/4 -> " 4"/1
  Demux/5 -> " 5"/1
  Demux/21 -> " 30"/1
  Demux/25 -> " 18"/1
  Demux/26 -> " 19"/1
  Demux/22 -> " 31"/1
  Demux/30 -> " 23"/1
  Demux/23 -> " 32"/1
  Demux/24 -> " 33"/1
  Demux/27 -> " 20"/1
  Demux/28 -> " 21"/1
  Demux/31 -> " 24"/1
  Demux/32 -> " 25"/1
  Demux/29 -> " 22"/1
  Demux/36 -> " 61"/1
  Demux/34 -> " 55"/1
  Demux/35 -> " 60"/1
  Demux/33 -> " 44"/1
  Demux/49 -> " 52"/1
  Demux/43 -> " 36"/1
  Demux/42 -> " 35"/1
  Demux/44 -> " 37"/1
  Demux/51 -> " 54"/1
  Demux/59 -> " 46"/1
  Demux/60 -> " 47"/1
  Demux/54 -> " 58"/1
  Demux/61 -> " 48"/1
  Demux/47 -> " 40"/1
  Demux/46 -> " 39"/1
  Demux/55 -> " 59"/1
  Demux/39 -> " 64"/1
  Demux/41 -> " 34"/1
  Demux/58 -> " 45"/1
  Demux/52 -> " 56"/1
  Demux/53 -> " 57"/1
  Demux/56 -> " 42"/1
  Demux/57 -> " 43"/1
  Demux/38 -> " 63"/1
  Demux/62 -> " 49"/1
  Demux/50 -> " 53"/1
  Demux/63 -> " 1"/1
  Demux/40 -> " 65"/1
  Demux/48 -> " 41"/1
  Demux/64 -> " 50"/1
  Demux/45 -> " 38"/1
  Demux/37 -> " 62"/1
  " 13"/1 -> Concat/13
  " 11"/1 -> Concat/11
  " 16"/1 -> Concat/16
  " 15"/1 -> Concat/15
  " 10"/1 -> Concat/10
  " 14"/1 -> Concat/14
  " 12"/1 -> Concat/12
  " 17"/1 -> Concat/17
  " 2"/1 -> Concat/2
  " 3"/1 -> Concat/3
  " 7"/1 -> Concat/7
  " 6"/1 -> Concat/6
  " 9"/1 -> Concat/9
  " 8"/1 -> Concat/8
  " 42"/1 -> Concat/56
  " 35"/1 -> Concat/42
  " 43"/1 -> Concat/57
  " 40"/1 -> Concat/47
  " 36"/1 -> Concat/43
  " 34"/1 -> Concat/41
  " 37"/1 -> Concat/44
  " 38"/1 -> Concat/45
  " 41"/1 -> Concat/48
  " 39"/1 -> Concat/46
  " 52"/1 -> Concat/49
  " 56"/1 -> Concat/52
  " 49"/1 -> Concat/62
  " 1"/1 -> Concat/63
  " 44"/1 -> Concat/33
  " 55"/1 -> Concat/34
  " 54"/1 -> Concat/51
  " 53"/1 -> Concat/50
  " 48"/1 -> Concat/61
  " 46"/1 -> Concat/59
  " 45"/1 -> Concat/58
  " 47"/1 -> Concat/60
  " 63"/1 -> Concat/38
  " 62"/1 -> Concat/37
  " 64"/1 -> Concat/39
  " 60"/1 -> Concat/35
  " 65"/1 -> Concat/40
  " 59"/1 -> Concat/55
  " 58"/1 -> Concat/54
  " 57"/1 -> Concat/53
  " 61"/1 -> Concat/36
  " 19"/1 -> Concat/26
  " 20"/1 -> Concat/27
  " 21"/1 -> Concat/28
  " 22"/1 -> Concat/29
  " 23"/1 -> Concat/30
  " 18"/1 -> Concat/25
  " 24"/1 -> Concat/31
  " 25"/1 -> Concat/32
  " 28"/1 -> Concat/19
  " 27"/1 -> Concat/18
  " 30"/1 -> Concat/21
  " 29"/1 -> Concat/20
  " 31"/1 -> Concat/22
  " 32"/1 -> Concat/23
  " 33"/1 -> Concat/24
  " 4"/1 -> Concat/4
  " 5"/1 -> Concat/5
  " 50"/1 -> Concat/64
  " 51"/1 -> Concat/1
  In1/1 -> Demux/1
  Concat/1 -> Out1/1

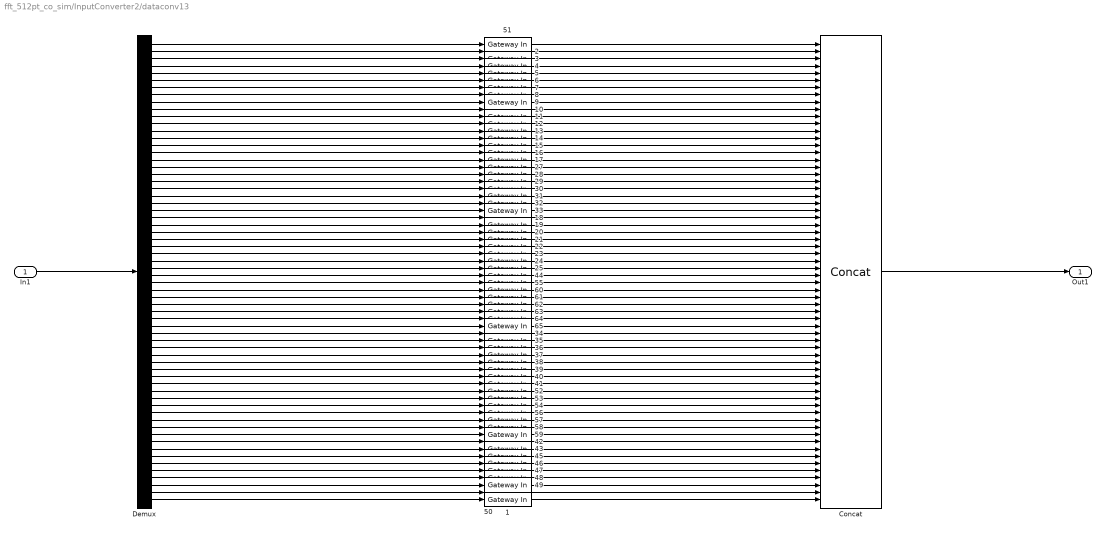
== system fft_512pt_co_sim/InputConverter2/dataconv13 ==
  In1 : Inport
   {1..25,27..65} (64 alike) : xbsIndex_r4/Gateway In  gui_display_data_type=Boolean  arith_type=Boolean  n_bits=16  bin_pt=14  preci_type=Single  exp_width=8  frac_width=24  quantization="Round  (unbiased: +/- Inf)"  overflow=Saturate  period=1  dbl_ovrd=off  timing_constraint=None  locs_specified=off  LOCs={}  UseAsADC=off  ADCChannel='1'  inherit_from_input=off  hdl_port=on  block_type=gatewayin
  Concat : xbsIndex_r4/Concat  num_inputs=64  dbl_ovrd=off  block_type=concat
  Demux : Demux  Outputs=64
  Out1 : Outport
  wires:
  Demux/12 -> " 12"/1
  Demux/14 -> " 14"/1
  Demux/15 -> " 15"/1
  Demux/17 -> " 17"/1
  Demux/10 -> " 10"/1
  Demux/16 -> " 16"/1
  Demux/18 -> " 27"/1
  Demux/19 -> " 28"/1
  Demux/7 -> " 7"/1
  Demux/20 -> " 29"/1
  Demux/9 -> " 9"/1
  Demux/2 -> " 2"/1
  Demux/13 -> " 13"/1
  Demux/3 -> " 3"/1
  Demux/6 -> " 6"/1
  Demux/11 -> " 11"/1
  Demux/1 -> " 51"/1
  Demux/8 -> " 8"/1
  Demux/4 -> " 4"/1
  Demux/5 -> " 5"/1
  Demux/21 -> " 30"/1
  Demux/25 -> " 18"/1
  Demux/26 -> " 19"/1
  Demux/22 -> " 31"/1
  Demux/30 -> " 23"/1
  Demux/23 -> " 32"/1
  Demux/24 -> " 33"/1
  Demux/27 -> " 20"/1
  Demux/28 -> " 21"/1
  Demux/31 -> " 24"/1
  Demux/32 -> " 25"/1
  Demux/29 -> " 22"/1
  Demux/36 -> " 61"/1
  Demux/34 -> " 55"/1
  Demux/35 -> " 60"/1
  Demux/33 -> " 44"/1
  Demux/49 -> " 52"/1
  Demux/43 -> " 36"/1
  Demux/42 -> " 35"/1
  Demux/44 -> " 37"/1
  Demux/51 -> " 54"/1
  Demux/59 -> " 46"/1
  Demux/60 -> " 47"/1
  Demux/54 -> " 58"/1
  Demux/61 -> " 48"/1
  Demux/47 -> " 40"/1
  Demux/46 -> " 39"/1
  Demux/55 -> " 59"/1
  Demux/39 -> " 64"/1
  Demux/41 -> " 34"/1
  Demux/58 -> " 45"/1
  Demux/52 -> " 56"/1
  Demux/53 -> " 57"/1
  Demux/56 -> " 42"/1
  Demux/57 -> " 43"/1
  Demux/38 -> " 63"/1
  Demux/62 -> " 49"/1
  Demux/50 -> " 53"/1
  Demux/63 -> " 1"/1
  Demux/40 -> " 65"/1
  Demux/48 -> " 41"/1
  Demux/64 -> " 50"/1
  Demux/45 -> " 38"/1
  Demux/37 -> " 62"/1
  " 13"/1 -> Concat/13
  " 11"/1 -> Concat/11
  " 16"/1 -> Concat/16
  " 15"/1 -> Concat/15
  " 10"/1 -> Concat/10
  " 14"/1 -> Concat/14
  " 12"/1 -> Concat/12
  " 17"/1 -> Concat/17
  " 2"/1 -> Concat/2
  " 3"/1 -> Concat/3
  " 7"/1 -> Concat/7
  " 6"/1 -> Concat/6
  " 9"/1 -> Concat/9
  " 8"/1 -> Concat/8
  " 42"/1 -> Concat/56
  " 35"/1 -> Concat/42
  " 43"/1 -> Concat/57
  " 40"/1 -> Concat/47
  " 36"/1 -> Concat/43
  " 34"/1 -> Concat/41
  " 37"/1 -> Concat/44
  " 38"/1 -> Concat/45
  " 41"/1 -> Concat/48
  " 39"/1 -> Concat/46
  " 52"/1 -> Concat/49
  " 56"/1 -> Concat/52
  " 49"/1 -> Concat/62
  " 1"/1 -> Concat/63
  " 44"/1 -> Concat/33
  " 55"/1 -> Concat/34
  " 54"/1 -> Concat/51
  " 53"/1 -> Concat/50
  " 48"/1 -> Concat/61
  " 46"/1 -> Concat/59
  " 45"/1 -> Concat/58
  " 47"/1 -> Concat/60
  " 63"/1 -> Concat/38
  " 62"/1 -> Concat/37
  " 64"/1 -> Concat/39
  " 60"/1 -> Concat/35
  " 65"/1 -> Concat/40
  " 59"/1 -> Concat/55
  " 58"/1 -> Concat/54
  " 57"/1 -> Concat/53
  " 61"/1 -> Concat/36
  " 19"/1 -> Concat/26
  " 20"/1 -> Concat/27
  " 21"/1 -> Concat/28
  " 22"/1 -> Concat/29
  " 23"/1 -> Concat/30
  " 18"/1 -> Concat/25
  " 24"/1 -> Concat/31
  " 25"/1 -> Concat/32
  " 28"/1 -> Concat/19
  " 27"/1 -> Concat/18
  " 30"/1 -> Concat/21
  " 29"/1 -> Concat/20
  " 31"/1 -> Concat/22
  " 32"/1 -> Concat/23
  " 33"/1 -> Concat/24
  " 4"/1 -> Concat/4
  " 5"/1 -> Concat/5
  " 50"/1 -> Concat/64
  " 51"/1 -> Concat/1
  In1/1 -> Demux/1
  Concat/1 -> Out1/1

== system fft_512pt_co_sim/InputConverter2/dataconv26 ==
  In1 : Inport
   {1..25,27..65} (64 alike) : xbsIndex_r4/Gateway In  gui_display_data_type=Boolean  arith_type=Boolean  n_bits=16  bin_pt=14  preci_type=Single  exp_width=8  frac_width=24  quantization="Round  (unbiased: +/- Inf)"  overflow=Saturate  period=1  dbl_ovrd=off  timing_constraint=None  locs_specified=off  LOCs={}  UseAsADC=off  ADCChannel='1'  inherit_from_input=off  hdl_port=on  block_type=gatewayin
  Concat : xbsIndex_r4/Concat  num_inputs=64  dbl_ovrd=off  block_type=concat
  Demux : Demux  Outputs=64
  Out1 : Outport
  wires:
  Demux/12 -> " 12"/1
  Demux/14 -> " 14"/1
  Demux/15 -> " 15"/1
  Demux/17 -> " 17"/1
  Demux/10 -> " 10"/1
  Demux/16 -> " 16"/1
  Demux/18 -> " 27"/1
  Demux/19 -> " 28"/1
  Demux/7 -> " 7"/1
  Demux/20 -> " 29"/1
  Demux/9 -> " 9"/1
  Demux/2 -> " 2"/1
  Demux/13 -> " 13"/1
  Demux/3 -> " 3"/1
  Demux/6 -> " 6"/1
  Demux/11 -> " 11"/1
  Demux/1 -> " 51"/1
  Demux/8 -> " 8"/1
  Demux/4 -> " 4"/1
  Demux/5 -> " 5"/1
  Demux/21 -> " 30"/1
  Demux/25 -> " 18"/1
  Demux/26 -> " 19"/1
  Demux/22 -> " 31"/1
  Demux/30 -> " 23"/1
  Demux/23 -> " 32"/1
  Demux/24 -> " 33"/1
  Demux/27 -> " 20"/1
  Demux/28 -> " 21"/1
  Demux/31 -> " 24"/1
  Demux/32 -> " 25"/1
  Demux/29 -> " 22"/1
  Demux/36 -> " 61"/1
  Demux/34 -> " 55"/1
  Demux/35 -> " 60"/1
  Demux/33 -> " 44"/1
  Demux/49 -> " 52"/1
  Demux/43 -> " 36"/1
  Demux/42 -> " 35"/1
  Demux/44 -> " 37"/1
  Demux/51 -> " 54"/1
  Demux/59 -> " 46"/1
  Demux/60 -> " 47"/1
  Demux/54 -> " 58"/1
  Demux/61 -> " 48"/1
  Demux/47 -> " 40"/1
  Demux/46 -> " 39"/1
  Demux/55 -> " 59"/1
  Demux/39 -> " 64"/1
  Demux/41 -> " 34"/1
  Demux/58 -> " 45"/1
  Demux/52 -> " 56"/1
  Demux/53 -> " 57"/1
  Demux/56 -> " 42"/1
  Demux/57 -> " 43"/1
  Demux/38 -> " 63"/1
  Demux/62 -> " 49"/1
  Demux/50 -> " 53"/1
  Demux/63 -> " 1"/1
  Demux/40 -> " 65"/1
  Demux/48 -> " 41"/1
  Demux/64 -> " 50"/1
  Demux/45 -> " 38"/1
  Demux/37 -> " 62"/1
  " 13"/1 -> Concat/13
  " 11"/1 -> Concat/11
  " 16"/1 -> Concat/16
  " 15"/1 -> Concat/15
  " 10"/1 -> Concat/10
  " 14"/1 -> Concat/14
  " 12"/1 -> Concat/12
  " 17"/1 -> Concat/17
  " 2"/1 -> Concat/2
  " 3"/1 -> Concat/3
  " 7"/1 -> Concat/7
  " 6"/1 -> Concat/6
  " 9"/1 -> Concat/9
  " 8"/1 -> Concat/8
  " 42"/1 -> Concat/56
  " 35"/1 -> Concat/42
  " 43"/1 -> Concat/57
  " 40"/1 -> Concat/47
  " 36"/1 -> Concat/43
  " 34"/1 -> Concat/41
  " 37"/1 -> Concat/44
  " 38"/1 -> Concat/45
  " 41"/1 -> Concat/48
  " 39"/1 -> Concat/46
  " 52"/1 -> Concat/49
  " 56"/1 -> Concat/52
  " 49"/1 -> Concat/62
  " 1"/1 -> Concat/63
  " 44"/1 -> Concat/33
  " 55"/1 -> Concat/34
  " 54"/1 -> Concat/51
  " 53"/1 -> Concat/50
  " 48"/1 -> Concat/61
  " 46"/1 -> Concat/59
  " 45"/1 -> Concat/58
  " 47"/1 -> Concat/60
  " 63"/1 -> Concat/38
  " 62"/1 -> Concat/37
  " 64"/1 -> Concat/39
  " 60"/1 -> Concat/35
  " 65"/1 -> Concat/40
  " 59"/1 -> Concat/55
  " 58"/1 -> Concat/54
  " 57"/1 -> Concat/53
  " 61"/1 -> Concat/36
  " 19"/1 -> Concat/26
  " 20"/1 -> Concat/27
  " 21"/1 -> Concat/28
  " 22"/1 -> Concat/29
  " 23"/1 -> Concat/30
  " 18"/1 -> Concat/25
  " 24"/1 -> Concat/31
  " 25"/1 -> Concat/32
  " 28"/1 -> Concat/19
  " 27"/1 -> Concat/18
  " 30"/1 -> Concat/21
  " 29"/1 -> Concat/20
  " 31"/1 -> Concat/22
  " 32"/1 -> Concat/23
  " 33"/1 -> Concat/24
  " 4"/1 -> Concat/4
  " 5"/1 -> Concat/5
  " 50"/1 -> Concat/64
  " 51"/1 -> Concat/1
  In1/1 -> Demux/1
  Concat/1 -> Out1/1
